simulink model "lambda"  (R2015b)
settings: Solver=FixedStepAuto  StartTime=0.0  StopTime=10.0  RelTol=1e-3
undefined symbols (not defined in the file or in its folder): tau_d_bc
settings Model: Creator=nicgr354  LastModifiedBy=nicgr354

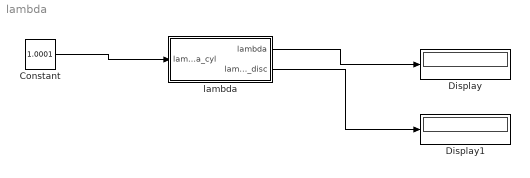
== system lambda ==
  Constant : Constant  Value=1.0001
  Display : Display
  Display1 : Display
      settings: Format=decimal (Stored Integer)
  lambda : Subsystem
  wires:
  Constant/1 -> lambda/1(lambda_cyl)
  lambda/1(lambda) -> Display/1
  lambda/2(lambda_bc_disc) -> Display1/1

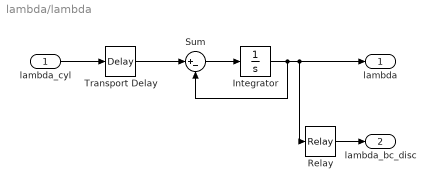
== system lambda/lambda ==
  lambda_cyl : Inport
  Integrator : Integrator
  Relay : Relay  OnSwitchValue=1  OffSwitchValue=1  OffOutputValue=-1
  Sum : Sum  Inputs=|+-
  Transport Delay : TransportDelay  DelayTime=tau_d_bc  InitialOutput=1
  lambda : Outport
  lambda_bc_disc : Outport  Port=2
  wires:
  lambda_cyl/1 -> Transport Delay/1
  Transport Delay/1 -> Sum/1
  Integrator/1 -> Sum/2, Relay/1, lambda/1
  Sum/1 -> Integrator/1
  Relay/1 -> lambda_bc_disc/1
